simulink model "engine_model_hierarchy"  (R2018a)
settings: Solver=VariableStepAuto  StartTime=0.0  StopTime=10.0  RelTol=1e-3
settings Model: Creator=Jarvis  LastModifiedBy=Jarvis

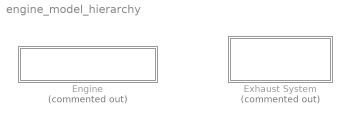
== system engine_model_hierarchy ==
  Engine : Subsystem  Commented=on
  "Exhaust System " : Subsystem  Commented=on

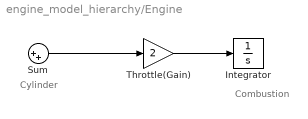
== system engine_model_hierarchy/Engine ==
  note: Combustion
  note: Cylinder
  Integrator : Integrator
  Sum : Sum  Inputs=|++
  Throttle(Gain) : Gain  Gain=2
  wires:
  Sum/1 -> Throttle(Gain)/1
  Throttle(Gain)/1 -> Integrator/1

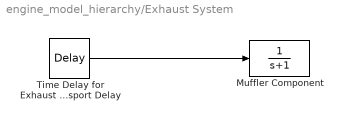
== system engine_model_hierarchy/Exhaust System  ==
  "Muffler Component " : TransferFcn  Denominator=[1 1]
  Time Delay for Exhaust simulated by Transport Delay : TransportDelay
  wires:
  Time Delay for Exhaust simulated by Transport Delay/1 -> "Muffler Component "/1
